simulink model "modelo8_comparacion"  (R2014a)
settings: Solver=ode15s  StartTime=0.0  StopTime=10  RelTol=1e-3
values from neighbouring files (symbols this model uses):
  A = [-2.0500   -0.4000         0         0         0         0 ... (first row only)    [matrices_ejemplo.m]
  B = [1.0000         0 ... (first row only)    [matrices_ejemplo.m]
  C = [0.0719   -0.5752   -0.1594    0.6378         0         0 ... (first row only)    [matrices_ejemplo.m]
  Kff = inv(R)*B'*inv((A-B*K)')*Q*L    [matrices_ejemplo.m]
undefined symbols (not defined in the file or in its folder): K, Kp
settings Model: Creator=Juan Pablo Requez  LastModifiedBy=Juan Pablo Requez
settings DataIOCC: LimitDataPoints=off  SaveFormat=Dataset
settings OptimizationCC: SimCompilerOptimization=off
settings DebuggingCC: MergeDetectMultiDrivingBlocksExec=error  SolverPrmCheckMsg=none  FrameProcessingCompatibilityMsg=error
settings HardwareCC: ProdBitPerPointer=64  ProdLargestAtomicFloat=Float  ProdIntDivRoundTo=Zero  ProdEndianess=LittleEndian  ProdWordSize=64  ProdHWDeviceType=Intel->x86-64 (Windows64)
settings ModelReferenceCC: PropagateSignalLabelsOutOfModel=on
settings RTWCC: RTWCompilerOptimization=off
settings ConfigComp: CovMetricSettings=dw  CovHtmlReporting=on  CovSaveCumulativeToWorkspaceVar=on  CovSaveSingleToWorkspaceVar=on  CovExternalEMLEnable=off

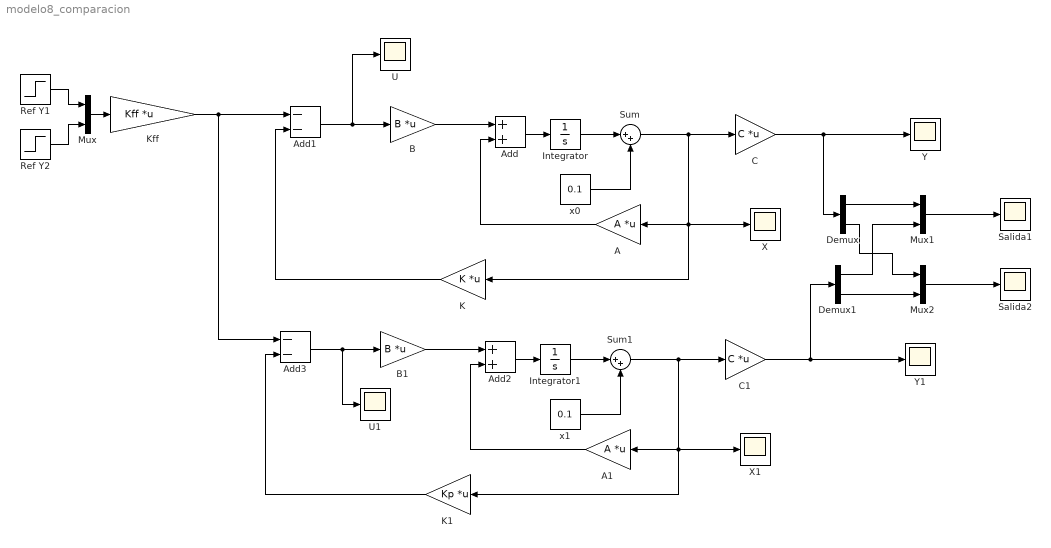
== system modelo8_comparacion ==
  A : Gain  Gain=A  Multiplication=Matrix(K*u)
  A1 : Gain  Gain=A  Multiplication=Matrix(K*u)
  Add : Sum
  Add1 : Sum  Inputs=--
  Add2 : Sum
  Add3 : Sum  Inputs=--
  B : Gain  Gain=B  Multiplication=Matrix(K*u)
  B1 : Gain  Gain=B  Multiplication=Matrix(K*u)
  C : Gain  Gain=C  Multiplication=Matrix(K*u)
  C1 : Gain  Gain=C  Multiplication=Matrix(K*u)
  Demux : Demux  Outputs=2
  Demux1 : Demux  Outputs=2
  Integrator : Integrator
  Integrator1 : Integrator
  K : Gain  Gain=K  Multiplication=Matrix(K*u)
  K1 : Gain  Gain=Kp  Multiplication=Matrix(K*u)
  Kff : Gain  Gain=Kff  Multiplication=Matrix(K*u)
  Mux : Mux  Inputs=2
  Mux1 : Mux  Inputs=2
  Mux2 : Mux  Inputs=2
  Ref Y1 : Step  Time=0  After=0  SampleTime=0
  Ref Y2 : Step  Time=0  After=0  SampleTime=0
  Salida1 : Scope
      settings: SaveName=Y2
  Salida2 : Scope
      settings: TimeRange=100  YMin=-0.15  YMax=0.04999999999999999  SaveName=Y3
  Sum : Sum  Inputs=|++
  Sum1 : Sum  Inputs=|++
  U : Scope
      settings: TimeRange=100  YMin=-2  YMax=0.5  SaveName=U
  U1 : Scope
      settings: TimeRange=100  YMin=-2  YMax=0.5  SaveName=U1
  X : Scope
      settings: SaveName=X
  X1 : Scope
      settings: SaveName=X1
  Y : Scope
      settings: SaveName=Y
  Y1 : Scope
      settings: SaveName=Y1
  x0 : Constant  Value=0.1
  x1 : Constant  Value=0.1
  wires:
  Add/1 -> Integrator/1
  B/1 -> Add/1
  A/1 -> Add/2
  Add1/1 -> U/1, B/1
  K/1 -> Add1/2
  C/1 -> Demux/1, Y/1
  Integrator/1 -> Sum/1
  Sum/1 -> K/1, A/1, X/1, C/1
  x0/1 -> Sum/2
  Mux/1 -> Kff/1
  Ref Y1/1 -> Mux/1
  Ref Y2/1 -> Mux/2
  Add2/1 -> Integrator1/1
  B1/1 -> Add2/1
  A1/1 -> Add2/2
  Add3/1 -> U1/1, B1/1
  K1/1 -> Add3/2
  Kff/1 -> Add3/1, Add1/1
  C1/1 -> Demux1/1, Y1/1
  Integrator1/1 -> Sum1/1
  Sum1/1 -> K1/1, A1/1, X1/1, C1/1
  x1/1 -> Sum1/2
  Demux/1 -> Mux1/1
  Demux1/1 -> Mux1/2
  Demux/2 -> Mux2/1
  Demux1/2 -> Mux2/2
  Mux1/1 -> Salida1/1
  Mux2/1 -> Salida2/1
